simulink model "carriersymbolpreamblesync"  (R2021a)
settings: Solver=ode45  StartTime=0.0  StopTime=inf  RelTol=1e-3  EnableMultiTasking=on
libraries: commsync2 x3, commdigbbndpm3 x2, commrandsrc3 x2, commfilt2 x2, commchan3 x1, commrfcorlib x1, commsink2 x1, commrflib2 x1, simulink x1, dspsigops x1
settings Model: Creator=The MathWorks, Inc.  LastModifiedBy=bruno
settings SolverCC: AlgebraicLoopSolver=TrustRegion
settings DataIOCC: LimitDataPoints=on  SaveFormat=Array  ReturnWorkspaceOutputs=off
settings OptimizationCC: LifeSpan=inf
settings DebuggingCC: SolverPrmCheckMsg=warning  AllowSymbolicDim=off  SFUnexpectedBacktrackingDiag=warning  SFNoUnconditionalDefaultTransitionDiag=warning  SFExecutionAtInitializationDiag=none  SFMachineParentedDataDiag=warning  ArithmeticOperatorsInVariantConditions=warning
settings HardwareCC: ProdBitPerPointer=32  ProdBitPerSizeT=32  ProdBitPerPtrDiffT=32  ProdLargestAtomicFloat=None  ProdIntDivRoundTo=Undefined  ProdEndianess=Unspecified  ProdWordSize=32  ProdHWDeviceType=32-bit Generic
settings ModelReferenceCC: PropagateSignalLabelsOutOfModel=off
settings SFSimCC: SimUseLocalCustomCode=off
settings RTWCC: RTWUseLocalCustomCode=off
settings CodeAppCC: StateflowObjectComments=on
settings GRTTargetCC: TargetLangStandard=C89/C90 (ANSI)
settings ConfigComp: CovMetricSettings=dw  CovSaveCumulativeToWorkspaceVar=on  CovSaveSingleToWorkspaceVar=on  CovExternalEMLEnable=off  CovSFcnEnable=off

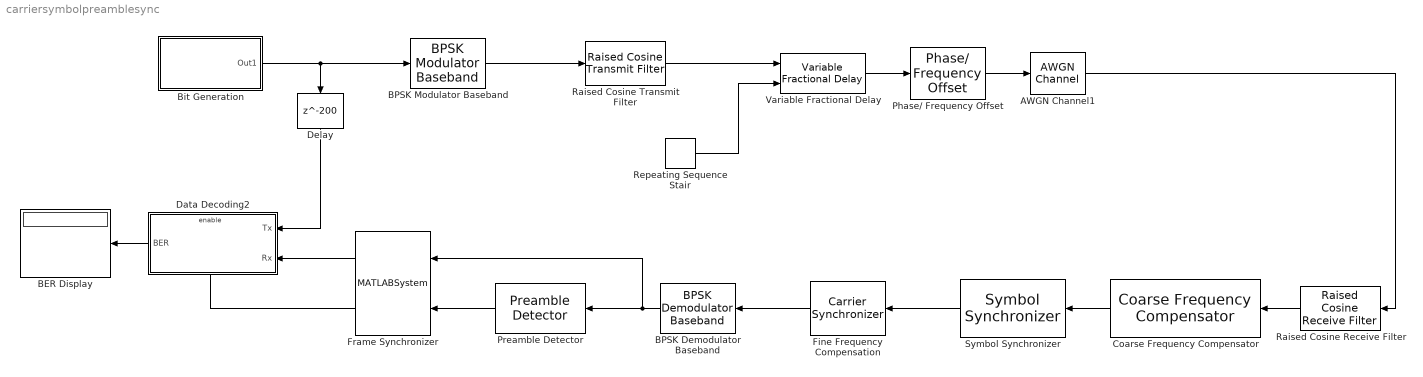
== system carriersymbolpreamblesync ==
  AWGN Channel1 : commchan3/AWGN Channel  InputProcessing=Columns as channels (frame based)  seed=67  noiseMode="Signal to noise ratio  (Eb/No)"  EbNodB=10  EsNodB=15  SNRdB=8  bitsPerSym=1  Ps=1/4  Tsym=1  variance=1
  BER Display : Display
  BPSK Demodulator Baseband : commdigbbndpm3/BPSK Demodulator Baseband  DecType=Hard decision  VarSource=Dialog  Variance=1  Ph=0  outDtype=Inherit via internal rule  derotateFactorWordLen=16  derotateFactorDataTypeStr=Inherit: Same word length as input  derotateFactorLastDataTypeStr=Inherit: Same word length as input
  BPSK Modulator Baseband : commdigbbndpm3/BPSK Modulator Baseband  Ph=0  outDtype=double  outWordLen=16  outUDDataType=sfix(16)  outFracLenMode=Best precision  outFracLen=15  outDataTypeStr=double  outLastDataTypeStr=double
  Bit Generation : Subsystem
      mask Display: disp('Bit Frame\nGeneration')
  Coarse Frequency Compensator : commrfcorlib/Coarse Frequency Compensator  Modulation=BPSK  Algorithm=FFT-based  FrequencyResolution=0.001  MaximumFrequencyOffset=0.05  SamplesPerSymbol=4  EstimatedFreqOffsetPort=off  SimulateUsing=Code generation
      settings: SourceProductBaseCode=CM
  Data Decoding2 : Subsystem
      mask Display: disp('Data Decoding');
  Delay : Delay  DelayLength=200  InputProcessing=Columns as channels (frame based)  UseCircularBuffer=on
  Fine Frequency Compensation : commsync2/Carrier Synchronizer  Modulation=BPSK  ModulationPhaseOffset=Auto  CustomPhaseOffset=0  SamplesPerSymbol=2  DampingFactor=1  NormalizedLoopBandwidth=0.01  EstimatedPhaseErrorOutputPort=off  SimulateUsing=Code generation
  Frame Synchronizer : MATLABSystem  System=comm.internal.examples.FrameSynchronizer  Input=Bit  OutputFrameLength=200  PreambleLength=40  SimulateUsing=Interpreted execution
      mask Type: comm.internal.examples.FrameSynchronizer
      mask Display:
      | disp(['Frame' char(10) 'Synchronizer']);
      | port_label('input',1,'u');
      | port_label('input',2,'idx');
      | port_label('output',1,'Frame');
      | port_label('output',2,'Valid');
  Phase/ Frequency Offset : commrflib2/Phase// Frequency Offset  phaseOffset=0  freqPort=off  freqOffset=10
  Preamble Detector : commsync2/Preamble Detector  Input=Bit  Preamble=[1 0 0 1 0 1 1 0 1 1 1 0 1 0 1 1 0 1 1 0 1 0 0 1 0 1 1 0 1 1 1 0 1 0 1 1 0 1 1 0]'  Threshold=3  DetectionMetricOutput=off  Detections=All  SimulateUsing=Interpreted execution
      settings: SourceProductBaseCode=CM
  Raised Cosine Receive Filter : commfilt2/Raised Cosine Receive Filter  filtType=Square root  R=0.5  filtSpan=10  N=4  downFactor=2  downOffset=0  filterGain=1  InputProcessing=Columns as channels (frame based)  RateOptions=Enforce single-rate processing  framing=Mute  checkCoeff=off  variableName=rcRxFilt  currentFiltSpan=10  D=(10)/2  inputOffset=0  sampMode=Mute  saveAsFlag=0  rateMode=Downsampling  checkGain=Normalized  launchFVT=on  roundingMode=Floor  overflowMode=off  coeffDataTypeStr=Inherit: Same word length as input  coeffMin=[]  coeffMax=[]  coeffLastDataTypeStr=Inherit: Same word length as input  accumDataTypeStr=Inherit: Same as product output  accumLastDataTypeStr=Inherit: Same as product output  outputDataTypeStr=Inherit: Same as accumulator  outputMin=[]  outputMax=[]  outputLastDataTypeStr=Inherit: Same as accumulator
  Raised Cosine Transmit Filter : commfilt2/Raised Cosine Transmit Filter  filtType=Square root  R=0.5  filtSpan=10  N=4  filterGain=1  InputProcessing=Columns as channels (frame based)  RateOptions=Enforce single-rate processing  framing=Mute  checkCoeff=off  variableName=rcTxFilt  checkGain=Normalized  sampMode=Mute  saveAsFlag=0  currentFiltSpan=10  D=(10)/2  launchFVT=on  roundingMode=Floor  overflowMode=off  coeffDataTypeStr=Inherit: Same word length as input  coeffMin=[]  coeffMax=[]  coeffLastDataTypeStr=Inherit: Same word length as input  outputDataTypeStr=Inherit: Same as accumulator  outputMin=[]  outputMax=[]  outputLastDataTypeStr=Inherit: Same as accumulator
  Repeating Sequence Stair : simulink/Sources/Repeating Sequence Stair  OutValues=[0:0.1:0.9 0.8:-0.1:0.1]  tsamp=-1  OutMin=[]  OutMax=[]  OutDataTypeStr=double  OutputDataTypeScalingMode=double  OutDataType=fixdt(0,8)  ConRadixGroup=Best Precision: Vector-wise  OutScaling=2^-12
  Symbol Synchronizer : commsync2/Symbol Synchronizer  Modulation=PAM/PSK/QAM  TimingErrorDetector=Early-Late (non-data-aided)  SamplesPerSymbol=2  DampingFactor=sqrt(2)/2  NormalizedLoopBandwidth=0.01  DetectorGain=2.7  TimingErrorOutputPort=off  SimulateUsing=Code generation
      settings: SourceProductBaseCode=CM
  Variable Fractional Delay : dspsigops/Variable Fractional Delay  mode=OBSOLETE  modeActive=Linear  L=4  FarrowL=4  R=10  alpha=1  dmax=400  InputProcessing=Columns as channels (frame based)  ic=0  noDFT=off  fallbackFIR=Clip to the minimum value necessary for centered kernel  fallbackFarrow=Clip to the minimum value necessary for centered kernel  roundingMode=Zero  overflowMode=off
      settings: SourceProductBaseCode=DS
  wires:
  BPSK Modulator Baseband/1 -> Raised Cosine Transmit Filter/1
  Bit Generation/1(Out1) -> BPSK Modulator Baseband/1, Delay/1
  AWGN Channel1/1 -> Raised Cosine Receive Filter/1
  Repeating Sequence Stair/1 -> Variable Fractional Delay/2
  Raised Cosine Transmit Filter/1 -> Variable Fractional Delay/1
  Variable Fractional Delay/1 -> Phase/ Frequency Offset/1
  Preamble Detector/1 -> Frame Synchronizer/2
  BPSK Demodulator Baseband/1 -> Frame Synchronizer/1, Preamble Detector/1
  Frame Synchronizer/1 -> Data Decoding2/2(Rx)
  Frame Synchronizer/2 -> Data Decoding2/Enable
  Delay/1 -> Data Decoding2/1(Tx)
  Data Decoding2/1(BER) -> BER Display/1
  Phase/ Frequency Offset/1 -> AWGN Channel1/1
  Raised Cosine Receive Filter/1 -> Coarse Frequency Compensator/1
  Symbol Synchronizer/1 -> Fine Frequency Compensation/1
  Fine Frequency Compensation/1 -> BPSK Demodulator Baseband/1
  Coarse Frequency Compensator/1 -> Symbol Synchronizer/1

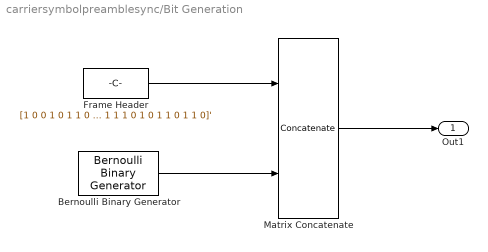
== system carriersymbolpreamblesync/Bit Generation ==
  Bernoulli Binary Generator : commrandsrc3/Bernoulli Binary Generator  ProbabilityOfZero=0.5  SeedSource=Parameter  Seed=61  SampleTime=1  SamplesPerFrame=160  OutputDataType=double  SimulateUsing=Interpreted execution
  Frame Header : Constant  Value=[1 0 0 1 0 1 1 0 1 1 1 0 1 0 1 1 0 1 1 0 1 0 0 1 0 1 1 0 1 1 1 0 1 0 1 1 0 1 1 0]'  VectorParams1D=off  OutDataTypeStr=double
  Matrix Concatenate : Concatenate  Mode=Multidimensional array
  Out1 : Outport  VectorParamsAs1DForOutWhenUnconnected=off
  wires:
  Matrix Concatenate/1 -> Out1/1
  Frame Header/1 -> Matrix Concatenate/1
  Bernoulli Binary Generator/1 -> Matrix Concatenate/2

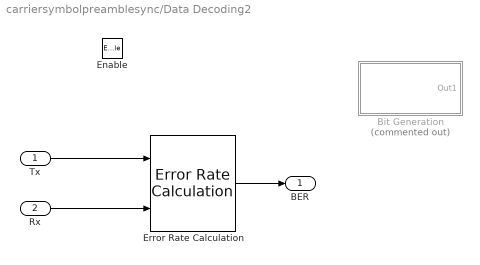
== system carriersymbolpreamblesync/Data Decoding2 ==
  Tx : Inport
  Rx : Inport  Port=2
  Enable : EnablePort
  Bit Generation : Subsystem  Commented=on
      mask Display: disp('Bit Frame\nGeneration')
  Error Rate Calculation : commsink2/Error Rate Calculation  N=0  st_delay=0  cp_mode=Entire frame  subframe=[]  PMode=Port  WsName=ErrorVec  RsMode2=off  stop=off  numErr=100  maxBits=1e6
  BER : Outport  VectorParamsAs1DForOutWhenUnconnected=off
  wires:
  Error Rate Calculation/1 -> BER/1
  Rx/1 -> Error Rate Calculation/2
  Tx/1 -> Error Rate Calculation/1

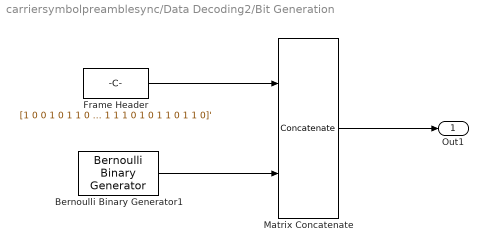
== system carriersymbolpreamblesync/Data Decoding2/Bit Generation ==
  Bernoulli Binary Generator1 : commrandsrc3/Bernoulli Binary Generator  ProbabilityOfZero=0.5  SeedSource=Parameter  Seed=61  SampleTime=1  SamplesPerFrame=160  OutputDataType=double  SimulateUsing=Interpreted execution
  Frame Header : Constant  Value=[1 0 0 1 0 1 1 0 1 1 1 0 1 0 1 1 0 1 1 0 1 0 0 1 0 1 1 0 1 1 1 0 1 0 1 1 0 1 1 0]'  VectorParams1D=off  OutDataTypeStr=double
  Matrix Concatenate : Concatenate  Mode=Multidimensional array
  Out1 : Outport  VectorParamsAs1DForOutWhenUnconnected=off
  wires:
  Matrix Concatenate/1 -> Out1/1
  Frame Header/1 -> Matrix Concatenate/1
  Bernoulli Binary Generator1/1 -> Matrix Concatenate/2
